simulink model "Battery_Motor"  (R2017b)
settings: Solver=VariableStepAuto  StartTime=0.0  StopTime=50  FixedStep=0.001  MaxStep=1e-4  RelTol=1e-4
values from neighbouring files (symbols this model uses):
  Amps = C/1000    (= 0.7)    [Battery_Dynamics.m]
  b_m = 2.415e-6    (= 2.415e-06)    [Battery_Dynamics.m]
  CD = 60    [Battery_Dynamics.m]
  Jr = 6.5*10^(-7)    (= 6.5e-07)    [Battery_Dynamics.m]
  Kemf = 0.00255    [Battery_Dynamics.m]
  Kt = Kemf    (= 0.00255)    [Battery_Dynamics.m]
  L = 0.001*R    (= 0.000117)    [Battery_Dynamics.m]
  PD = 120    [Battery_Dynamics.m]
  R = 0.117    [Battery_Dynamics.m]
undefined symbols (not defined in the file or in its folder): Ion, Lithium
libraries: simulink x4, powerlib x2, electricdrivelib x1, dspstat3 x1
settings Model: Creator=Nicky  LastModifiedBy=Nicky
settings SolverCC: ZeroCrossAlgorithm=Adaptive  AutoInsertRateTranBlk=on
settings DebuggingCC: MaxConsecutiveZCsMsg=none
settings CodeAppCC: StateflowObjectComments=on
settings SimscapeCC: SimscapeNormalizeSystem=off

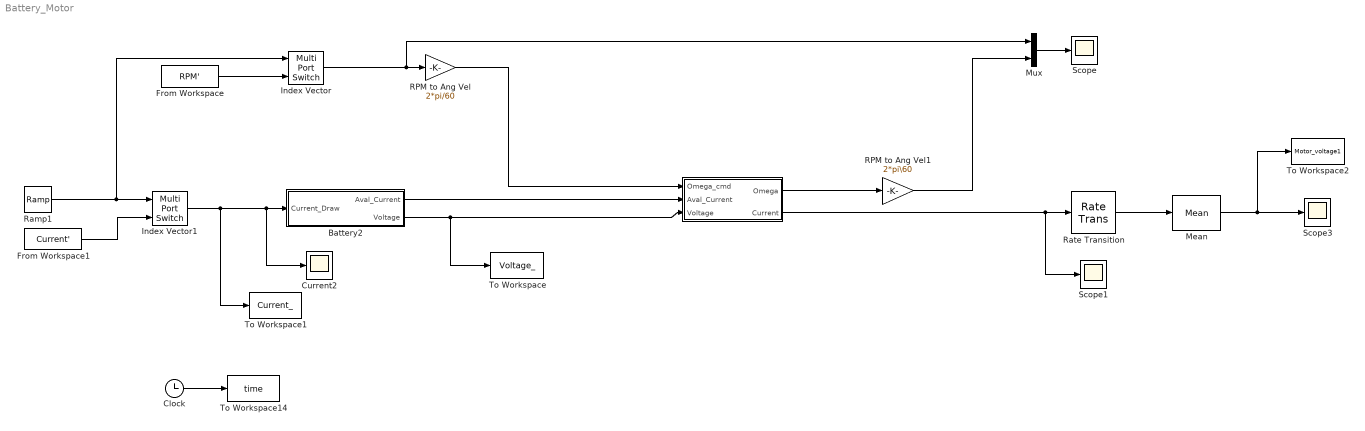
== system Battery_Motor ==
  " " : Subsystem
  Battery2 : Subsystem
  Clock : Clock
  Current2 : Scope
  From Workspace : FromWorkspace  VariableName=RPM'  OutDataTypeStr=double
  From Workspace1 : FromWorkspace  VariableName=Current'  OutDataTypeStr=double
  Index Vector : MultiPortSwitch  DataPortOrder=Zero-based contiguous  Inputs=1  zeroidx=on
  Index Vector1 : MultiPortSwitch  DataPortOrder=Zero-based contiguous  Inputs=1  zeroidx=on
  Mean : dspstat3/Mean  run=on  reset_popup=None  InputProcessing=Columns as channels (frame based)  directionMode=Each column  dimension=1  roiEnable=off  roiType=Rectangles  roiPortion=Entire ROI  roiOutput=Individual statistics for each ROI  roiFlag=off  outputDataTypeStr=Inherit: Same as accumulator  outputLastDataTypeStr=Inherit: Same as accumulator  outputMin=[]  outputMax=[]  roundingMode=Floor  overflowMode=off
  Mux : Mux  Inputs=2
  RPM to Ang Vel : Gain  Gain=2*pi/60
  RPM to Ang Vel1 : Gain  Gain=2*pi\60
  Ramp1 : simulink/Sources/Ramp  slope=100  start=0  X0=1
  Rate Transition : RateTransition  OutPortSampleTime=0.001
  Scope : Scope
  Scope1 : Scope
  Scope3 : Scope
  To Workspace : ToWorkspace  VariableName=Voltage_  SampleTime=0.001
      settings: Save2DSignal=2-D array (concatenate along first dimension)
  To Workspace1 : ToWorkspace  VariableName=Current_  SampleTime=0.001
      settings: Save2DSignal=2-D array (concatenate along first dimension)
  To Workspace14 : ToWorkspace  VariableName=time  SampleTime=0.001
      settings: Save2DSignal=2-D array (concatenate along first dimension)
  To Workspace2 : ToWorkspace  VariableName=Motor_voltage1  SampleTime=0.001
      settings: Save2DSignal=2-D array (concatenate along first dimension)
  wires:
  RPM to Ang Vel/1 -> " "/1(Omega_cmd)
  " "/1(Omega) -> RPM to Ang Vel1/1
  From Workspace/1 -> Index Vector/2
  Index Vector/1 -> Mux/1, RPM to Ang Vel/1
  From Workspace1/1 -> Index Vector1/2
  Index Vector1/1 -> To Workspace1/1, Current2/1, Battery2/1(Current_Draw)
  Clock/1 -> To Workspace14/1
  Battery2/2(Voltage) -> To Workspace/1, " "/3(Voltage)
  Ramp1/1 -> Index Vector/1, Index Vector1/1
  Battery2/1(Aval_Current) -> " "/2(Aval_Current)
  Mux/1 -> Scope/1
  RPM to Ang Vel1/1 -> Mux/2
  Mean/1 -> Scope3/1, To Workspace2/1
  " "/2("Current ") -> Scope1/1, Rate Transition/1
  Rate Transition/1 -> Mean/1

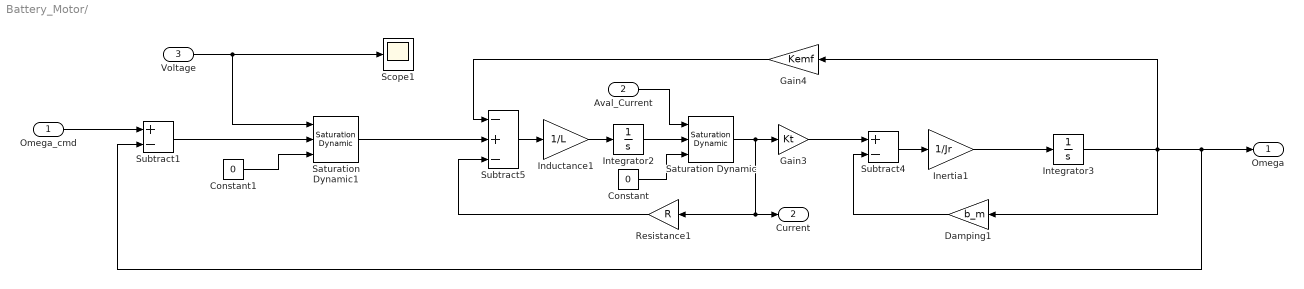
== system Battery_Motor/  ==
  Omega_cmd : Inport
  Aval_Current : Inport  Port=2
  Voltage : Inport  Port=3
  Constant : Constant  Value=0
  Constant1 : Constant  Value=0
  Damping1 : Gain  Gain=b_m
  Gain3 : Gain  Gain=Kt
  Gain4 : Gain  Gain=Kemf
  Inductance1 : Gain  Gain=1/L
  Inertia1 : Gain  Gain=1/Jr
  Integrator2 : Integrator  LimitOutput=on  LowerSaturationLimit=0
  Integrator3 : Integrator  LimitOutput=on  LowerSaturationLimit=0
  Resistance1 : Gain  Gain=R
  Saturation Dynamic : simulink/Discontinuities/Saturation Dynamic  OutMin=[]  OutMax=[]  OutDataTypeStr=Inherit: Same as second input  OutDataType=fixdt(1, 16)  OutScaling=2^-10  DoSatur=off
  Saturation Dynamic1 : simulink/Discontinuities/Saturation Dynamic  OutMin=[]  OutMax=[]  OutDataTypeStr=Inherit: Same as second input  OutDataType=fixdt(1, 16)  OutScaling=2^-10  DoSatur=off
  Scope1 : Scope
  Subtract1 : Sum  Inputs=+-
  Subtract4 : Sum  Inputs=+-
  Subtract5 : Sum  Inputs=-+-
  Omega : Outport
  "Current " : Outport  Port=2
  wires:
  Inertia1/1 -> Integrator3/1
  Resistance1/1 -> Subtract5/3
  Damping1/1 -> Subtract4/2
  Subtract5/1 -> Inductance1/1
  Saturation Dynamic1/1 -> Subtract5/2
  Gain4/1 -> Subtract5/1
  Subtract4/1 -> Inertia1/1
  Gain3/1 -> Subtract4/1
  Omega_cmd/1 -> Subtract1/1
  Integrator3/1 -> Damping1/1, Subtract1/2, Omega/1, Gain4/1
  Inductance1/1 -> Integrator2/1
  Aval_Current/1 -> Saturation Dynamic/1
  Constant/1 -> Saturation Dynamic/3
  Saturation Dynamic/1 -> Resistance1/1, "Current "/1, Gain3/1
  Integrator2/1 -> Saturation Dynamic/2
  Voltage/1 -> Scope1/1, Saturation Dynamic1/1
  Constant1/1 -> Saturation Dynamic1/3
  Subtract1/1 -> Saturation Dynamic1/2

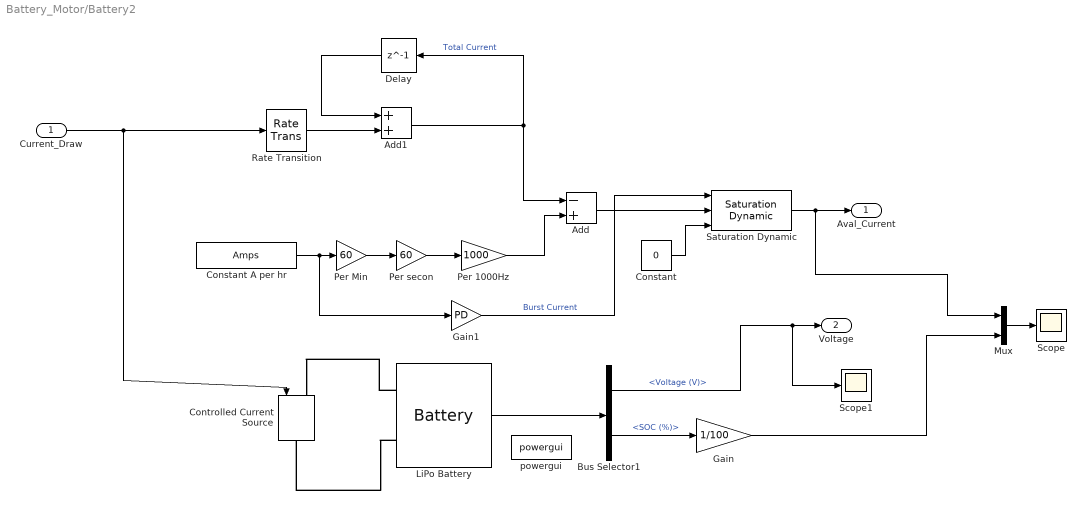
== system Battery_Motor/Battery2 ==
  Current_Draw : Inport
  Add : Sum  Inputs=-+
  Add1 : Sum
  Bus Selector1 : BusSelector  OutputSignals=Voltage (V),SOC (%)
  Constant : Constant  Value=0
  Constant A per hr : Constant  Value=Amps
  Controlled Current Source : powerlib/Electrical Sources/Controlled Current Source  Initialize=on  Source_Type=DC  Amplitude=0  Phase=0  Frequency=0  Measurements=None
  Delay : Delay  DelayLength=1  InitialCondition=0
  Gain : Gain  Gain=1/100
  Gain1 : Gain  Gain=PD
  "LiPo Battery " : electricdrivelib/Extra Sources/Battery  BatType=Lithium-Ion  ShowTempParam=off  ThermalPreset=no  ShowAgeParam=off  NomV=11.1  NomQ=.7  SOC=100  Batt_Tr=1  PresetModel=off  MaxQ=0.7  MinV=8.325  FullV=11.7  Dis_rate=.7  R=.11  Normal_OP=.7  expZone="[11.7   0.5]"  current=CD*Amps  Units=Ampere-hour  Tci=20  NomT=25  T2=0  MaxQ2=2.208  FullV2=3.45  Normal_OP2=2.8  expZone2="[3.22        0.23]"  Rca=0.6  ti=1000  Dp=0  Neq0=0  Tsim=1e6  Ta1=25  Qeol=5.4*0.9  Reol=0.013333*1.2  Char_age=[2.3478, 3]  Dis_age=[2.3478, 10]  N1=1500  N2=10500  N3=1000  N4=1400  Ta2=45  N5=950
  Mux : Mux  Inputs=2
  Per 1000Hz : Gain  Gain=1000
  Per Min : Gain  Gain=60
  Per secon : Gain  Gain=60
  Rate Transition : RateTransition  OutPortSampleTimeMultiple=0  OutPortSampleTime=0.001
  Saturation Dynamic : simulink/Discontinuities/Saturation Dynamic  OutMin=[]  OutMax=[]  OutDataTypeStr=Inherit: Same as second input  OutDataType=fixdt(1, 16)  OutScaling=2^-10  DoSatur=off
  Scope : Scope
  Scope1 : Scope
  powergui : powerlib/powergui  SimulationMode=Continuous  SampleTime=0.001  frequency=60  Iterations=50  frequencyindice=0  Pbase=100e6  ErrMax=1e-4  UnitsV=kV  UnitsW=MW  buscounter=0  FunctionMessages=off  echomessages=off  EnableUseOfTLC=off  CurrentSourceSwitches=off  DisableSnubberDevices=off  DisableRonSwitches=off  DisableVfSwitches=off  DisplayEquations=off  SolverType=Tustin/Backward Euler (TBE)  Interpol=off  ExternalGateDelay=off  methode=off  Ts=100  x0status=blocks  SPID=on  SwTol=0  HookPort=off  RestoreLinks=warning  ResistiveCurrentMeasurement=off  Frange=[0:2:500]  Ylog=off  Xlog=on  ShowGrid=off  save=off  variable=ZData  structure=0  ZoomFFT=on  StartTime=0.0  cycles=1  DisplayStyle=1  fundamental=60  FreqAxis=off  MaxFrequency=1000  frequencyindicesteady=1  RmsSteady=1  display=off
  Aval_Current : Outport
  Voltage : Outport  Port=2
  wires:
  Per Min/1 -> Per secon/1
  Constant A per hr/1 -> Gain1/1, Per Min/1
  Per secon/1 -> Per 1000Hz/1
  Per 1000Hz/1 -> Add/2
  Add1/1 -> Add/1, Delay/1  "Total Current"
  Rate Transition/1 -> Add1/2
  Delay/1 -> Add1/1
  Constant/1 -> Saturation Dynamic/3
  Bus Selector1/1 -> Scope1/1, Voltage/1  "<Voltage (V)>"
  Bus Selector1/2 -> Gain/1  "<SOC (%)>"
  Gain/1 -> Mux/2
  "LiPo Battery "/1 -> Bus Selector1/1
  Add/1 -> Saturation Dynamic/2
  Gain1/1 -> Saturation Dynamic/1  "Burst Current"
  Saturation Dynamic/1 -> Mux/1, Aval_Current/1
  Mux/1 -> Scope/1
  Current_Draw/1 -> Controlled Current Source/1, Rate Transition/1
  connections:
  "LiPo Battery "/LConn1 -- Controlled Current Source/LConn1
  "LiPo Battery "/LConn2 -- Controlled Current Source/RConn1
